simulink subsystem "DAC_SubSystem"  (R2020b)
settings: Solver=VariableStepAuto  StartTime=0.0  StopTime=10.0  RelTol=1e-3
values from neighbouring files (symbols this model uses):
  Ts = T2    (= 0.01)    [PIDAntiWindupDigital.m]    (also in PIDDigital.m = 0.001; StateSpaceControllerNominalCont.m = 0.001; StateSpaceControllerNominalDigital.m = 0.001; StateSpaceControllerNominalDirectDigital.m = 0.05)
settings Model: Creator=umberto  LastModifiedBy=umbe

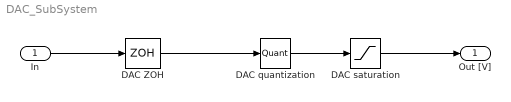
== system DAC_SubSystem ==
  In : Inport
  DAC ZOH : ZeroOrderHold  SampleTime=Ts
  DAC quantization : Quantizer  QuantizationInterval=20/(2^(16) - 1)
  DAC saturation : Saturate  UpperLimit=10  LowerLimit=-10
  Out [V] : Outport
  wires:
  DAC saturation/1 -> Out [V]/1
  DAC quantization/1 -> DAC saturation/1
  DAC ZOH/1 -> DAC quantization/1
  In/1 -> DAC ZOH/1
